simulink subsystem "proc_nav_ros_input"  (R2025b)
settings: Solver=VariableStepAuto  StartTime=0.0  StopTime=10.0  RelTol=1e-3
undefined symbols (not defined in the file): config, simulink
libraries: ros2lib x23, simulink x4
settings Model: Creator=relat  LastModifiedBy=ubuntu

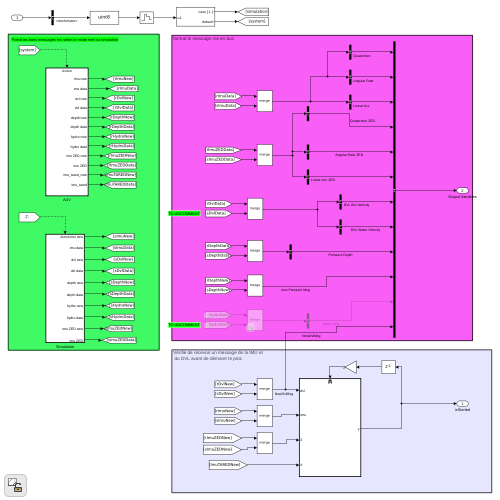
[thumbnail: Simulink's stored preview of the top-level diagram]
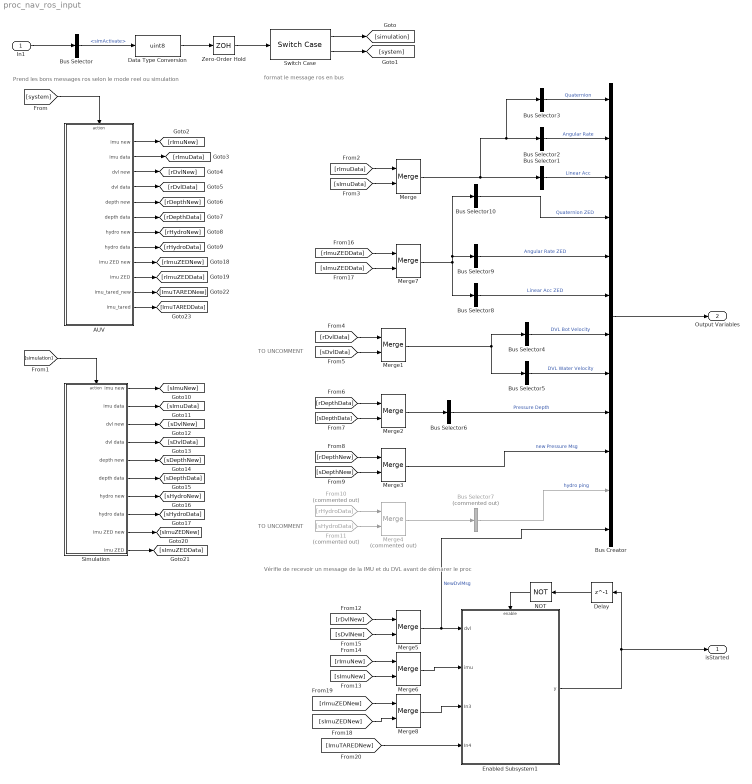
== system proc_nav_ros_input ==
  note: Vérifie de recevoir un message de la IMU et
      |  du DVL avant de démarer le proc
  note: format le message ros en bus
  note: TO UNCOMMENT
  note: Prend les bons messages ros selon le mode reel ou simulation
  note: TO UNCOMMENT
  In1 : Inport
  AUV : Subsystem  TreatAsAtomicUnit=on
  Bus Creator : BusCreator  Inputs=12
  Bus Selector : BusSelector  OutputSignals=simActivate
  Bus Selector1 : BusSelector  OutputSignals=linear_acceleration  OutputAsBus=on
  Bus Selector10 : BusSelector  OutputSignals=orientation.w,orientation.x,orientation.y,orientation.z  OutputAsBus=on
  Bus Selector2 : BusSelector  OutputSignals=angular_velocity  OutputAsBus=on
  Bus Selector3 : BusSelector  OutputSignals=orientation.w,orientation.x,orientation.y,orientation.z  OutputAsBus=on
  Bus Selector4 : BusSelector  OutputSignals=x_vel_btm,y_vel_btm,z_vel_btm,e_vel_btm  OutputAsBus=on
  Bus Selector5 : BusSelector  OutputSignals=velocity1,velocity2,velocity3,velocity4  OutputAsBus=on
  Bus Selector6 : BusSelector  OutputSignals=data  OutputAsBus=on
  Bus Selector7 : BusSelector  Commented=on  OutputSignals=heading,elevation  OutputAsBus=on
  Bus Selector8 : BusSelector  OutputSignals=linear_acceleration  OutputAsBus=on
  Bus Selector9 : BusSelector  OutputSignals=angular_velocity  OutputAsBus=on
  Data Type Conversion : DataTypeConversion  OutDataTypeStr=uint8  SaturateOnIntegerOverflow=off  RndMeth=Floor
  Delay : Delay  DelayLength=1  InitialCondition=0
  Enabled Subsystem1 : Subsystem  TreatAsAtomicUnit=on
  From10 : From  Commented=on  GotoTag=rHydroData
  From11 : From  Commented=on  GotoTag=sHydroData
  Merge{,1..3,5..8} (8 alike) : Merge
  Merge4 : Merge  Commented=on
  NOT : Logic  Operator=NOT  IconShape=distinctive  AllPortsSameDT=off  OutDataTypeStr=boolean
  Simulation : Subsystem  TreatAsAtomicUnit=on
  Switch Case : SwitchCase
  Zero-Order Hold : ZeroOrderHold  SampleTime=simulink.procNav.sampletime
  isStarted : Outport
  Output Variables : Outport  Port=2
  wires:
  In1/1 -> Bus Selector/1
  Bus Selector/1 -> Data Type Conversion/1  "<simActivate>"
  Data Type Conversion/1 -> Zero-Order Hold/1
  Zero-Order Hold/1 -> Switch Case/1
  Switch Case/1 -> [simulation]
  Switch Case/2 -> [system]
  [system] -> AUV/Action
  AUV/1(imu new) -> [rImuNew]
  AUV/2(imu data) -> [rImuData]
  AUV/3(dvl new) -> [rDvlNew]
  AUV/4(dvl data) -> [rDvlData]
  AUV/5(depth new) -> [rDepthNew]
  AUV/6(depth data) -> [rDepthData]
  AUV/7(hydro new) -> [rHydroNew]
  AUV/8(hydro data) -> [rHydroData]
  Simulation/5(depth new) -> [sDepthNew]
  Simulation/4(dvl data) -> [sDvlData]
  Simulation/7(hydro new) -> [sHydroNew]
  Simulation/2(imu data) -> [sImuData]
  Simulation/1(imu new) -> [sImuNew]
  [simulation] -> Simulation/Action
  Simulation/6(depth data) -> [sDepthData]
  Simulation/3(dvl new) -> [sDvlNew]
  Simulation/8(hydro data) -> [sHydroData]
  [rImuData] -> Merge/1
  [sImuData] -> Merge/2
  Merge/1 -> Bus Selector1/1, Bus Selector2/1, Bus Selector3/1
  [rDvlData] -> Merge1/1
  [sDvlData] -> Merge1/2
  [sDepthData] -> Merge2/2
  [rDepthData] -> Merge2/1
  Merge2/1 -> Bus Selector6/1
  [rDepthNew] -> Merge3/1
  [sDepthNew] -> Merge3/2
  From10/1 -> Merge4/1
  From11/1 -> Merge4/2
  Bus Selector3/1 -> Bus Creator/1  "Quaternion"
  Bus Selector2/1 -> Bus Creator/2  "Angular Rate"
  Bus Selector1/1 -> Bus Creator/3  "Linear Acc"
  Bus Selector4/1 -> Bus Creator/7  "DVL Bot Velocity"
  Bus Selector5/1 -> Bus Creator/8  "DVL Water Velocity"
  Bus Selector6/1 -> Bus Creator/9  "Pressure Depth"
  Merge3/1 -> Bus Creator/10  "new Pressure Msg"
  [rImuNew] -> Merge6/1
  Delay/1 -> NOT/1
  Bus Creator/1 -> Output Variables/1
  Merge1/1 -> Bus Selector5/1, Bus Selector4/1
  [sImuNew] -> Merge6/2
  Simulation/10(imu ZED) -> [sImuZEDData]
  Simulation/9(imu ZED new) -> [sImuZEDNew]
  AUV/10(imu ZED) -> [rImuZEDData]
  AUV/9(imu ZED new) -> [rImuZEDNew]
  [rImuZEDData] -> Merge7/1
  Bus Selector8/1 -> Bus Creator/6  "Linear Acc ZED"
  [sImuZEDData] -> Merge7/2
  Merge7/1 -> Bus Selector9/1, Bus Selector10/1, Bus Selector8/1
  Bus Selector10/1 -> Bus Creator/4  "Quaternion ZED"
  Bus Selector9/1 -> Bus Creator/5  "Angular Rate ZED"
  Merge4/1 -> Bus Selector7/1
  Bus Selector7/1 -> Bus Creator/11  "hydro ping"
  Enabled Subsystem1/1(y) -> isStarted/1, Delay/1
  Merge6/1 -> Enabled Subsystem1/2(imu)
  NOT/1 -> Enabled Subsystem1/Enable
  Merge8/1 -> Enabled Subsystem1/3(In3)
  [sDvlNew] -> Merge5/2
  Merge5/1 -> Enabled Subsystem1/1(dvl), Bus Creator/12  "NewDvlMsg"
  [rDvlNew] -> Merge5/1
  [rImuZEDNew] -> Merge8/1
  [sImuZEDNew] -> Merge8/2
  AUV/12(imu_tared) -> [ImuTAREDData]
  AUV/11(imu_tared_new) -> [ImuTAREDNew]
  [ImuTAREDNew] -> Enabled Subsystem1/4(In4)

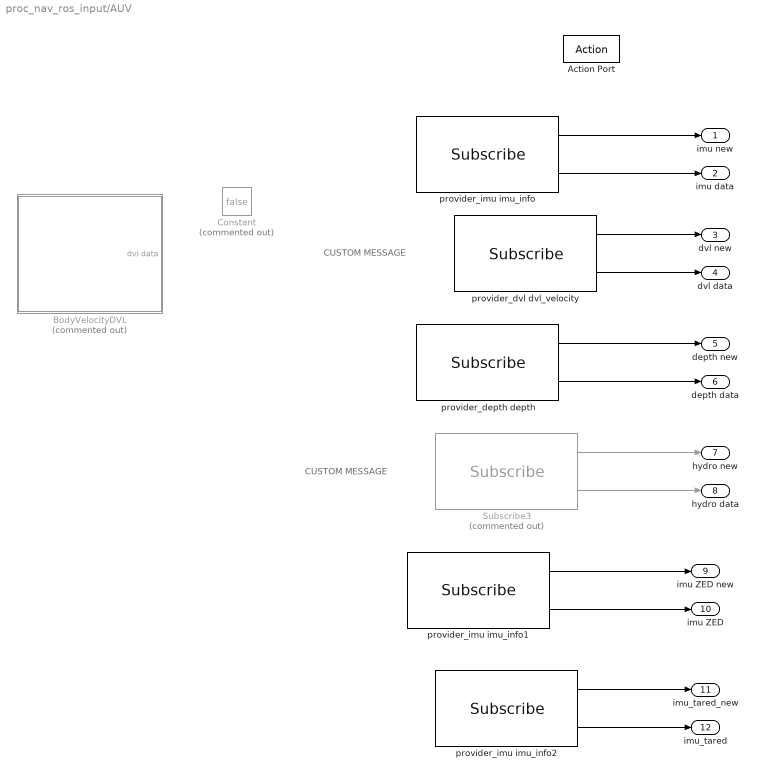
== system proc_nav_ros_input/AUV ==
  note: CUSTOM MESSAGE
  note: CUSTOM MESSAGE
  Action Port : ActionPort
  BodyVelocityDVL : Subsystem  Commented=on
  Constant : Constant  Commented=on  Value=false  VectorParams1D=off  SampleTime=-1
  Subscribe3 : ros2lib/Subscribe  Commented=on  topicSource=Specify your own  topic=/proc_hydro/ping  messageType=sonia_common_ros2/PingAngles  sampleTime=simulink.procNav.sampletime  QOSHistory=Keep last  QOSDepth=1  QOSReliability=Reliable  QOSDurability=Volatile  QOSDeadline=5  QOSLifespan=5  QOSLiveliness=Automatic  QOSLeaseDuration=5  QOSAvoidROSNamespaceConventions=off
  provider_depth depth : ros2lib/Subscribe  topicSource=Specify your own  topic=/provider_depth/depth  messageType=std_msgs/Float32  sampleTime=simulink.procNav.sampletime  QOSHistory=Keep last  QOSDepth=10  QOSReliability=Reliable  QOSDurability=Volatile  QOSDeadline=inf  QOSLifespan=inf  QOSLiveliness=Automatic  QOSLeaseDuration=inf  QOSAvoidROSNamespaceConventions=off
  provider_dvl dvl_velocity : ros2lib/Subscribe  topicSource=Specify your own  topic=/provider_dvl/dvl_velocity  messageType=sonia_common_ros2/BodyVelocityDVL  sampleTime=simulink.procNav.sampletime  QOSHistory=Keep last  QOSDepth=10  QOSReliability=Reliable  QOSDurability=Volatile  QOSDeadline=inf  QOSLifespan=inf  QOSLiveliness=Automatic  QOSLeaseDuration=inf  QOSAvoidROSNamespaceConventions=off
  provider_imu imu_info : ros2lib/Subscribe  topicSource=Specify your own  topic=/provider_imu/imu_info  messageType=sensor_msgs/Imu  sampleTime=simulink.procNav.sampletime  QOSHistory=Keep last  QOSDepth=10  QOSReliability=Reliable  QOSDurability=Volatile  QOSDeadline=inf  QOSLifespan=inf  QOSLiveliness=Automatic  QOSLeaseDuration=inf  QOSAvoidROSNamespaceConventions=off
  provider_imu imu_info1 : ros2lib/Subscribe  topicSource=Specify your own  topic=/zed/zed_node/imu/data  messageType=sensor_msgs/Imu  sampleTime=simulink.procNav.sampletime  QOSHistory=Keep last  QOSDepth=10  QOSReliability=Reliable  QOSDurability=Volatile  QOSDeadline=inf  QOSLifespan=inf  QOSLiveliness=Automatic  QOSLeaseDuration=inf  QOSAvoidROSNamespaceConventions=off
  provider_imu imu_info2 : ros2lib/Subscribe  topicSource=Specify your own  topic=/proc_control/imu_tared  messageType=std_msgs/Bool  sampleTime=simulink.procNav.sampletime  QOSHistory=Keep last  QOSDepth=10  QOSReliability=Reliable  QOSDurability=Volatile  QOSDeadline=inf  QOSLifespan=inf  QOSLiveliness=Automatic  QOSLeaseDuration=inf  QOSAvoidROSNamespaceConventions=off
  imu new : Outport
  imu data : Outport  Port=2
  dvl new : Outport  Port=3
  dvl data : Outport  Port=4
  depth new : Outport  Port=5
  depth data : Outport  Port=6
  hydro new : Outport  Port=7
  hydro data : Outport  Port=8
  imu ZED new : Outport  Port=9
  imu ZED : Outport  Port=10
  imu_tared_new : Outport  Port=11
  imu_tared : Outport  Port=12
  wires:
  provider_imu imu_info2/1 -> imu_tared_new/1
  provider_imu imu_info2/2 -> imu_tared/1
  provider_imu imu_info1/1 -> imu ZED new/1
  provider_imu imu_info1/2 -> imu ZED/1
  provider_dvl dvl_velocity/2 -> dvl data/1
  provider_depth depth/2 -> depth data/1
  provider_depth depth/1 -> depth new/1
  provider_dvl dvl_velocity/1 -> dvl new/1
  Subscribe3/1 -> hydro new/1
  Subscribe3/2 -> hydro data/1
  provider_imu imu_info/1 -> imu new/1
  provider_imu imu_info/2 -> imu data/1

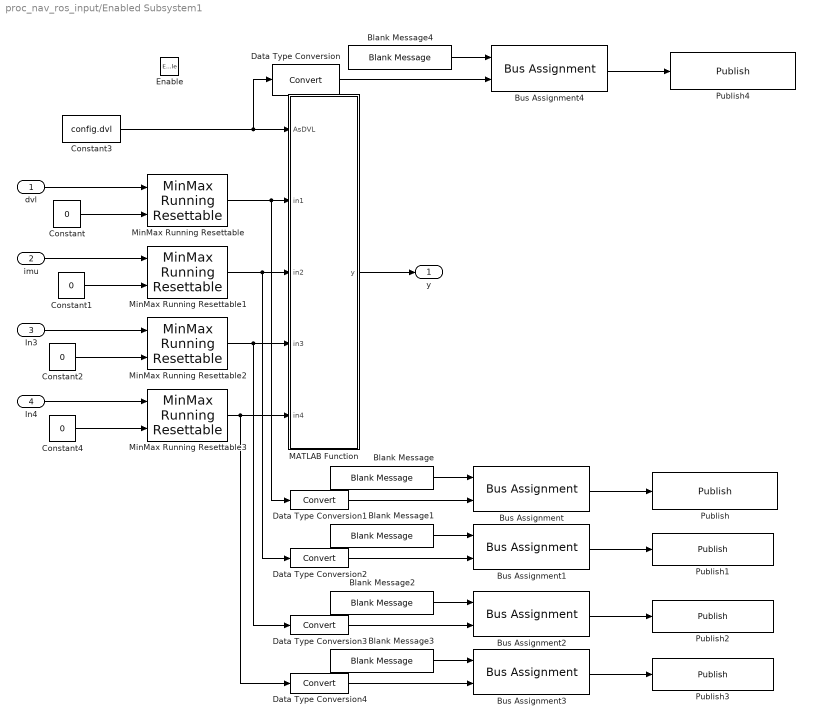
== system proc_nav_ros_input/Enabled Subsystem1 ==
  dvl : Inport
  imu : Inport  Port=2
  In3 : Inport  Port=3
  In4 : Inport  Port=4
  Enable : EnablePort
  Blank Message{,1..4} (5 alike) : ros2lib/Blank Message  messageClass=Message  entityType=std_msgs/Bool  messageType=std_msgs/Bool  SampleTime=inf
  Bus Assignment{,1..4} (5 alike) : BusAssignment  AssignedSignals=data
  Constant{,1..2,4} (4 alike) : Constant  Value=0
  Constant3 : Constant  Value=config.dvl
  Data Type Conversion{,1..4} (5 alike) : DataTypeConversion  SaturateOnIntegerOverflow=off  RndMeth=Floor
  MATLAB Function : MATLAB Function  TreatAsAtomicUnit=on
  MinMax Running Resettable{,1..3} (4 alike) : simulink/Math Operations/MinMax Running Resettable  Function=max  vinit=0.0
  Publish : ros2lib/Publish  topicSource=Specify your own  topic=/proc_control/dvl_enable  messageType=std_msgs/Bool  QOSHistory=Keep last  QOSDepth=1  QOSReliability=Reliable  QOSDurability=Volatile  QOSDeadline=Inf  QOSLifespan=Inf  QOSLiveliness=Automatic  QOSLeaseDuration=Inf  QOSAvoidROSNamespaceConventions=off
  Publish1 : ros2lib/Publish  topicSource=Specify your own  topic=/proc_control/imu_enable  messageType=std_msgs/Bool  QOSHistory=Keep last  QOSDepth=1  QOSReliability=Reliable  QOSDurability=Volatile  QOSDeadline=Inf  QOSLifespan=Inf  QOSLiveliness=Automatic  QOSLeaseDuration=Inf  QOSAvoidROSNamespaceConventions=off
  Publish2 : ros2lib/Publish  topicSource=Specify your own  topic=/proc_control/zed_enable  messageType=std_msgs/Bool  QOSHistory=Keep last  QOSDepth=1  QOSReliability=Reliable  QOSDurability=Volatile  QOSDeadline=Inf  QOSLifespan=Inf  QOSLiveliness=Automatic  QOSLeaseDuration=Inf  QOSAvoidROSNamespaceConventions=off
  Publish3 : ros2lib/Publish  topicSource=Specify your own  topic=/proc_control/imu_tared  messageType=std_msgs/Bool  QOSHistory=Keep last  QOSDepth=1  QOSReliability=Reliable  QOSDurability=Volatile  QOSDeadline=Inf  QOSLifespan=Inf  QOSLiveliness=Automatic  QOSLeaseDuration=Inf  QOSAvoidROSNamespaceConventions=off
  Publish4 : ros2lib/Publish  topicSource=Specify your own  topic=/proc_control/dvl_enable  messageType=std_msgs/Bool  QOSHistory=Keep last  QOSDepth=1  QOSReliability=Reliable  QOSDurability=Volatile  QOSDeadline=Inf  QOSLifespan=Inf  QOSLiveliness=Automatic  QOSLeaseDuration=Inf  QOSAvoidROSNamespaceConventions=off
  y : Outport
  wires:
  Blank Message4/1 -> Bus Assignment4/1
  Bus Assignment4/1 -> Publish4/1
  Blank Message3/1 -> Bus Assignment3/1
  Bus Assignment3/1 -> Publish3/1
  Bus Assignment2/1 -> Publish2/1
  Blank Message2/1 -> Bus Assignment2/1
  Blank Message1/1 -> Bus Assignment1/1
  Bus Assignment1/1 -> Publish1/1
  Bus Assignment/1 -> Publish/1
  Blank Message/1 -> Bus Assignment/1
  MATLAB Function/1(y) -> y/1
  Constant2/1 -> MinMax Running Resettable2/2
  Constant4/1 -> MinMax Running Resettable3/2
  imu/1 -> MinMax Running Resettable1/1
  Constant1/1 -> MinMax Running Resettable1/2
  Constant/1 -> MinMax Running Resettable/2
  dvl/1 -> MinMax Running Resettable/1
  In3/1 -> MinMax Running Resettable2/1
  In4/1 -> MinMax Running Resettable3/1
  Constant3/1 -> MATLAB Function/1(AsDVL), Data Type Conversion/1
  Data Type Conversion/1 -> Bus Assignment4/2
  MinMax Running Resettable/1 -> MATLAB Function/2(in1), Data Type Conversion1/1
  Data Type Conversion1/1 -> Bus Assignment/2
  MinMax Running Resettable1/1 -> MATLAB Function/3(in2), Data Type Conversion2/1
  Data Type Conversion2/1 -> Bus Assignment1/2
  MinMax Running Resettable2/1 -> MATLAB Function/4(in3), Data Type Conversion3/1
  Data Type Conversion3/1 -> Bus Assignment2/2
  MinMax Running Resettable3/1 -> MATLAB Function/5(in4), Data Type Conversion4/1
  Data Type Conversion4/1 -> Bus Assignment3/2

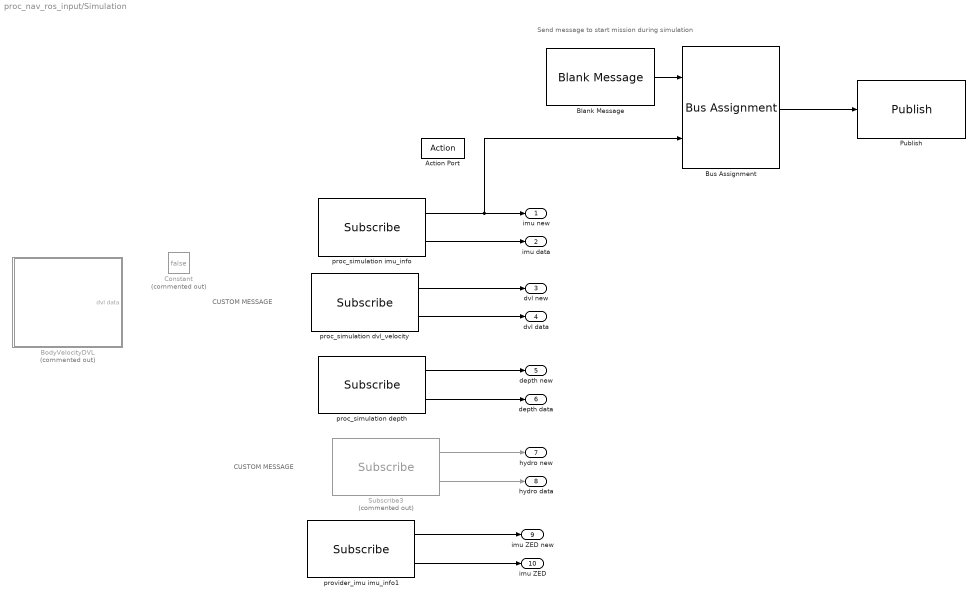
== system proc_nav_ros_input/Simulation ==
  note: CUSTOM MESSAGE
  note: CUSTOM MESSAGE
  note: Send message to start mission during simulation
  Action Port : ActionPort
  Blank Message : ros2lib/Blank Message  messageClass=Message  entityType=std_msgs/Bool  messageType=std_msgs/Bool  SampleTime=inf
  BodyVelocityDVL : Subsystem  Commented=on
  Bus Assignment : BusAssignment  AssignedSignals=data
  Constant : Constant  Commented=on  Value=false  VectorParams1D=off
  Publish : ros2lib/Publish  topicSource=Specify your own  topic=/proc_simulation/in_simulation  messageType=std_msgs/Bool  QOSHistory=Keep last  QOSDepth=1  QOSReliability=Reliable  QOSDurability=Volatile  QOSDeadline=Inf  QOSLifespan=Inf  QOSLiveliness=Automatic  QOSLeaseDuration=Inf  QOSAvoidROSNamespaceConventions=off
  Subscribe3 : ros2lib/Subscribe  Commented=on  topicSource=Specify your own  topic=/proc_simulation/ping  messageType=sonia_common_ros2/PingAngles  sampleTime=simulink.procNav.sampletime  QOSHistory=Keep last  QOSDepth=1  QOSReliability=Reliable  QOSDurability=Volatile  QOSDeadline=5  QOSLifespan=5  QOSLiveliness=Automatic  QOSLeaseDuration=5  QOSAvoidROSNamespaceConventions=off
  proc_simulation depth : ros2lib/Subscribe  topicSource=Specify your own  topic=/proc_simulation/depth  messageType=std_msgs/Float32  sampleTime=simulink.procNav.sampletime  QOSHistory=Keep last  QOSDepth=10  QOSReliability=Reliable  QOSDurability=Volatile  QOSDeadline=inf  QOSLifespan=inf  QOSLiveliness=Automatic  QOSLeaseDuration=inf  QOSAvoidROSNamespaceConventions=off
  proc_simulation dvl_velocity : ros2lib/Subscribe  topicSource=Specify your own  topic=/proc_simulation/dvl_velocity  messageType=sonia_common_ros2/BodyVelocityDVL  sampleTime=simulink.procNav.sampletime  QOSHistory=Keep last  QOSDepth=10  QOSReliability=Reliable  QOSDurability=Volatile  QOSDeadline=inf  QOSLifespan=inf  QOSLiveliness=Automatic  QOSLeaseDuration=inf  QOSAvoidROSNamespaceConventions=off
  proc_simulation imu_info : ros2lib/Subscribe  topicSource=Specify your own  topic=/proc_simulation/imu_info  messageType=sensor_msgs/Imu  sampleTime=simulink.procNav.sampletime  QOSHistory=Keep last  QOSDepth=10  QOSReliability=Reliable  QOSDurability=Volatile  QOSDeadline=inf  QOSLifespan=inf  QOSLiveliness=Automatic  QOSLeaseDuration=inf  QOSAvoidROSNamespaceConventions=off
  provider_imu imu_info1 : ros2lib/Subscribe  topicSource=Specify your own  topic=/proc_simulation/imu/data  messageType=sensor_msgs/Imu  sampleTime=simulink.procNav.sampletime  QOSHistory=Keep last  QOSDepth=10  QOSReliability=Reliable  QOSDurability=Volatile  QOSDeadline=inf  QOSLifespan=inf  QOSLiveliness=Automatic  QOSLeaseDuration=inf  QOSAvoidROSNamespaceConventions=off
  imu new : Outport
  imu data : Outport  Port=2
  dvl new : Outport  Port=3
  dvl data : Outport  Port=4
  depth new : Outport  Port=5
  depth data : Outport  Port=6
  hydro new : Outport  Port=7
  hydro data : Outport  Port=8
  imu ZED new : Outport  Port=9
  imu ZED : Outport  Port=10
  wires:
  Bus Assignment/1 -> Publish/1
  Blank Message/1 -> Bus Assignment/1
  proc_simulation dvl_velocity/2 -> dvl data/1
  proc_simulation depth/2 -> depth data/1
  proc_simulation depth/1 -> depth new/1
  proc_simulation dvl_velocity/1 -> dvl new/1
  proc_simulation imu_info/2 -> imu data/1
  proc_simulation imu_info/1 -> imu new/1, Bus Assignment/2
  Subscribe3/1 -> hydro new/1
  Subscribe3/2 -> hydro data/1
  provider_imu imu_info1/1 -> imu ZED new/1
  provider_imu imu_info1/2 -> imu ZED/1

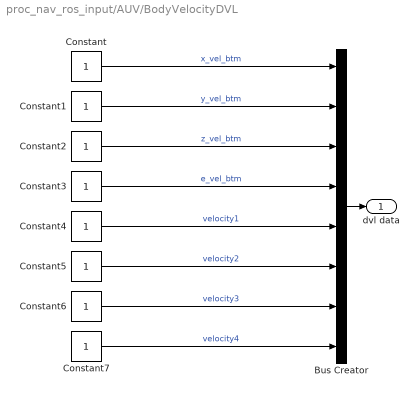
== system proc_nav_ros_input/AUV/BodyVelocityDVL ==
  Bus Creator : BusCreator  Inputs=8
  Constant{,1..7} (8 alike) : Constant  SampleTime=-1
  dvl data : Outport
  wires:
  Constant/1 -> Bus Creator/1  "x_vel_btm"
  Constant4/1 -> Bus Creator/5  "velocity1"
  Constant6/1 -> Bus Creator/7  "velocity3"
  Constant3/1 -> Bus Creator/4  "e_vel_btm"
  Constant5/1 -> Bus Creator/6  "velocity2"
  Bus Creator/1 -> dvl data/1
  Constant7/1 -> Bus Creator/8  "velocity4"
  Constant1/1 -> Bus Creator/2  "y_vel_btm"
  Constant2/1 -> Bus Creator/3  "z_vel_btm"

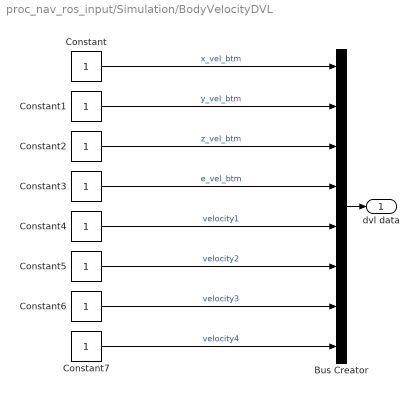
== system proc_nav_ros_input/Simulation/BodyVelocityDVL ==
  Bus Creator : BusCreator  Inputs=8
  Constant{,1..7} (8 alike) : Constant
  dvl data : Outport
  wires:
  Constant/1 -> Bus Creator/1  "x_vel_btm"
  Constant4/1 -> Bus Creator/5  "velocity1"
  Constant6/1 -> Bus Creator/7  "velocity3"
  Constant3/1 -> Bus Creator/4  "e_vel_btm"
  Constant5/1 -> Bus Creator/6  "velocity2"
  Bus Creator/1 -> dvl data/1
  Constant7/1 -> Bus Creator/8  "velocity4"
  Constant1/1 -> Bus Creator/2  "y_vel_btm"
  Constant2/1 -> Bus Creator/3  "z_vel_btm"

== matlab function proc_nav_ros_input/Enabled Subsystem1/MATLAB Function ==
  data: AsDVL input; in1 input; y output; in2 input; in3 input; in4 input
function y = fcn(AsDVL, in1,in2, in3, in4)

    if AsDVL && in1+in2+in3+in4 >=4
        y=1;
    elseif in2+in3+in4 >=3
        y=1;
    else
        y=0;
    end
end
